simulink model "ACsystem"  (R2023b)
settings: Solver=VariableStepAuto  StartTime=0.0  StopTime=10.0  RelTol=1e-3
settings Model: Creator=elija  LastModifiedBy=elija

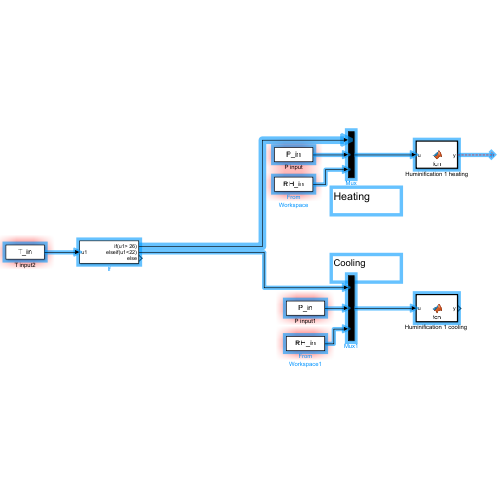
[thumbnail: Simulink's stored preview of the top-level diagram]
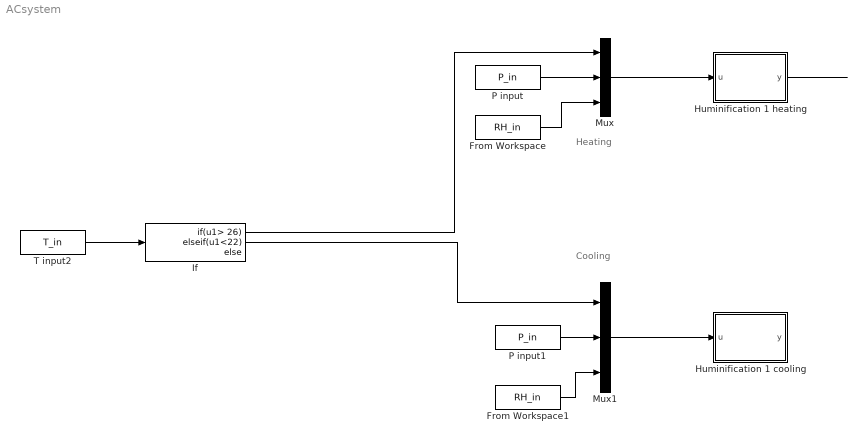
== system ACsystem ==
  note: Heating
  note: Cooling
  From Workspace : FromWorkspace  VariableName=RH_in
  From Workspace1 : FromWorkspace  VariableName=RH_in
  "Huminification 1 cooling " : MATLAB Function  TreatAsAtomicUnit=on
  Huminification 1 heating : MATLAB Function  TreatAsAtomicUnit=on
  If : If  IfExpression=u1> 26  ElseIfExpressions=u1<22
  Mux : Mux  Inputs=3
  Mux1 : Mux  Inputs=3
  P input : FromWorkspace  VariableName=P_in
  P input1 : FromWorkspace  VariableName=P_in
  T input2 : FromWorkspace  VariableName=T_in
  wires:
  T input2/1 -> If/1
  P input/1 -> Mux/2
  From Workspace/1 -> Mux/3
  If/1 -> Mux/1
  If/2 -> Mux1/1
  P input1/1 -> Mux1/2
  From Workspace1/1 -> Mux1/3
  Mux/1 -> Huminification 1 heating/1(u)
  Huminification 1 heating/1(y) -> ?
  Mux1/1 -> "Huminification 1 cooling "/1(u)

== matlab function ACsystem/Huminification 1 heating ==
  data: u input; y output
function y = fcn(u)

y = u;

== matlab function ACsystem/Huminification 1 cooling  ==
  data: u input; y output
function y = fcn(u)

y = u;
